simulink model "Induction_Machine_Model1"  (Simulink 7.5)
settings: Solver=ode45  StartTime=0.0  StopTime=0.2  MaxStep=0.001  RelTol=1e-3
settings Model: Creator=CN  LastModifiedBy=pradhyumna
settings DebuggingCC: StrictBusMsg=Warning

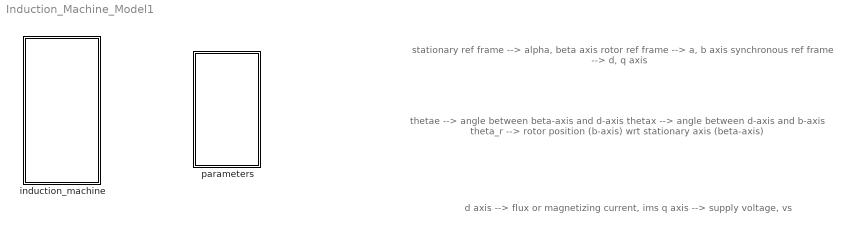
== system Induction_Machine_Model1 ==
  note: thetae --> angle between beta-axis and d-axis
      | thetax --> angle between d-axis and b-axis
      | theta_r --> rotor position (b-axis) wrt stationary axis (beta-axis)
  note: stationary ref frame --> alpha, beta axis
      | rotor ref frame --> a, b axis
      | synchronous ref frame --> d, q axis
  note: d axis --> flux or magnetizing current, ims
      | q axis --> supply voltage, vs
  induction_machine : Subsystem
  parameters : Subsystem

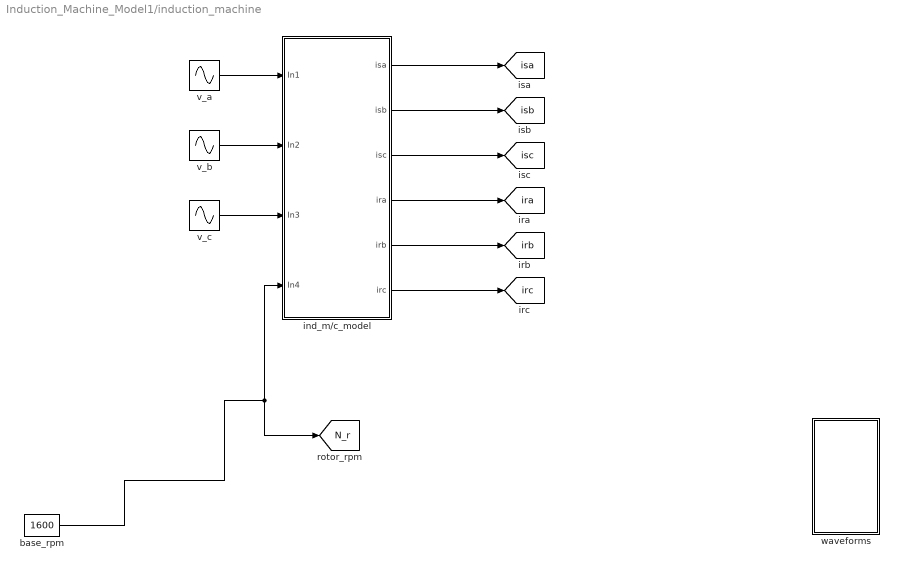
== system Induction_Machine_Model1/induction_machine ==
  base_rpm : Constant  Value=1600  OutDataType=sfix(16)  OutScaling=2^0
  ind_m/c_model : Subsystem
  v_a : Sin  Amplitude=239.6*sqrt(2)  Bias=0  Frequency=2*pi*50  Phase=0  Samples=10  SampleTime=0  Offset=0
  v_b : Sin  Amplitude=239.6*sqrt(2)  Bias=0  Frequency=2*pi*50  Phase=-2*pi/3  Samples=10  SampleTime=0  Offset=0
  v_c : Sin  Amplitude=239.6*sqrt(2)  Bias=0  Frequency=2*pi*50  Phase=-4*pi/3  Samples=10  SampleTime=0  Offset=0
  waveforms : Subsystem
  tag scope: N_r=global, ira=global, irb=global, irc=global, isa=global, isb=global, isc=global
  wires:
  ind_m/c_model/6(irc) -> [irc]
  ind_m/c_model/5(irb) -> [irb]
  ind_m/c_model/4(ira) -> [ira]
  ind_m/c_model/3(isc) -> [isc]
  ind_m/c_model/2(isb) -> [isb]
  ind_m/c_model/1(isa) -> [isa]
  v_c/1 -> ind_m/c_model/3(In3)
  v_b/1 -> ind_m/c_model/2(In2)
  v_a/1 -> ind_m/c_model/1(In1)
  base_rpm/1 -> ind_m/c_model/4(In4), [N_r]

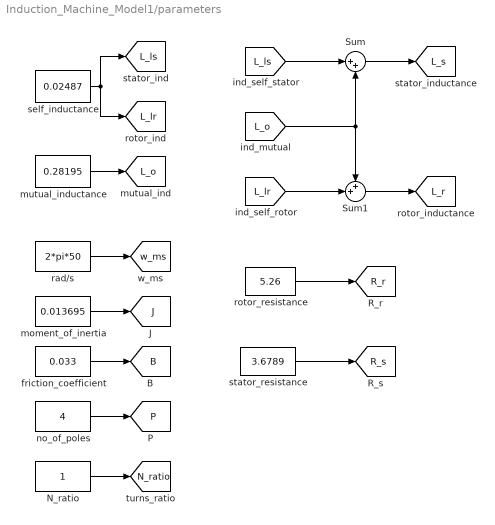
== system Induction_Machine_Model1/parameters ==
  N_ratio : Constant  OutDataType=sfix(16)  OutScaling=2^0
  Sum : Sum  Inputs=|++  OutDataType=sfix(16)  OutScaling=2^0
  Sum1 : Sum  Inputs=++|  OutDataType=sfix(16)  OutScaling=2^0
  friction_coefficient : Constant  Value=0.033  OutDataType=sfix(16)  OutScaling=2^0
  moment_of_inertia : Constant  Value=0.013695  OutDataType=sfix(16)  OutScaling=2^0
  mutual_inductance : Constant  Value=0.28195  OutDataType=sfix(16)  OutScaling=2^0
  no_of_poles : Constant  Value=4  OutDataType=sfix(16)  OutScaling=2^0
  rad/s : Constant  Value=2*pi*50  OutDataType=sfix(16)  OutScaling=2^0
  rotor_resistance : Constant  Value=5.26  OutDataType=sfix(16)  OutScaling=2^0
  self_inductance : Constant  Value=0.02487  OutDataType=sfix(16)  OutScaling=2^0
  stator_resistance : Constant  Value=3.6789  OutDataType=sfix(16)  OutScaling=2^0
  tag scope: B=global, J=global, L_lr=global, L_ls=global, L_o=global, L_r=global, L_s=global, N_ratio=global, P=global, R_r=global, R_s=global, w_ms=global
  wires:
  self_inductance/1 -> [L_ls], [L_lr]
  rad/s/1 -> [w_ms]
  moment_of_inertia/1 -> [J]
  friction_coefficient/1 -> [B]
  no_of_poles/1 -> [P]
  N_ratio/1 -> [N_ratio]
  [L_lr] -> Sum1/2
  [L_ls] -> Sum/1
  Sum/1 -> [L_s]
  Sum1/1 -> [L_r]
  rotor_resistance/1 -> [R_r]
  mutual_inductance/1 -> [L_o]
  stator_resistance/1 -> [R_s]
  [L_o] -> Sum/2, Sum1/1

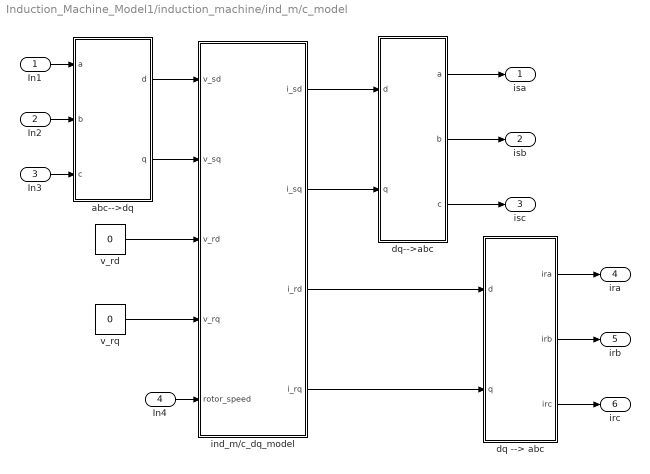
== system Induction_Machine_Model1/induction_machine/ind_m/c_model ==
  In1 : Inport  OutDataType=sfix(16)  OutScaling=2^0
  In2 : Inport  Port=2  OutDataType=sfix(16)  OutScaling=2^0
  In3 : Inport  Port=3  OutDataType=sfix(16)  OutScaling=2^0
  In4 : Inport  Port=4  OutDataType=sfix(16)  OutScaling=2^0
  abc-->dq : Subsystem
  dq --> abc : Subsystem
  dq-->abc : Subsystem
  ind_m/c_dq_model : Subsystem
  v_rd : Constant  Value=0  OutDataType=fixdt(1, 16)  OutScaling=2^0
  v_rq : Constant  Value=0  OutDataType=fixdt(1, 16)  OutScaling=2^0
  isa : Outport  OutDataType=sfix(16)  OutScaling=2^0
  isb : Outport  Port=2  OutDataType=sfix(16)  OutScaling=2^0
  isc : Outport  Port=3  OutDataType=sfix(16)  OutScaling=2^0
  ira : Outport  Port=4  OutDataType=sfix(16)  OutScaling=2^0
  irb : Outport  Port=5  OutDataType=sfix(16)  OutScaling=2^0
  irc : Outport  Port=6  OutDataType=sfix(16)  OutScaling=2^0
  wires:
  ind_m/c_dq_model/1(i_sd) -> dq-->abc/1(d)
  ind_m/c_dq_model/2(i_sq) -> dq-->abc/2(q)
  abc-->dq/2(q) -> ind_m/c_dq_model/2(v_sq)
  abc-->dq/1(d) -> ind_m/c_dq_model/1(v_sd)
  ind_m/c_dq_model/3(i_rd) -> dq --> abc/1(d)
  ind_m/c_dq_model/4(i_rq) -> dq --> abc/2(q)
  In1/1 -> abc-->dq/1(a)
  dq-->abc/1(a) -> isa/1
  In2/1 -> abc-->dq/2(b)
  dq-->abc/2(b) -> isb/1
  In3/1 -> abc-->dq/3(c)
  dq-->abc/3(c) -> isc/1
  dq --> abc/1(ira) -> ira/1
  dq --> abc/2(irb) -> irb/1
  dq --> abc/3(irc) -> irc/1
  In4/1 -> ind_m/c_dq_model/5(rotor_speed)
  v_rd/1 -> ind_m/c_dq_model/3(v_rd)
  v_rq/1 -> ind_m/c_dq_model/4(v_rq)

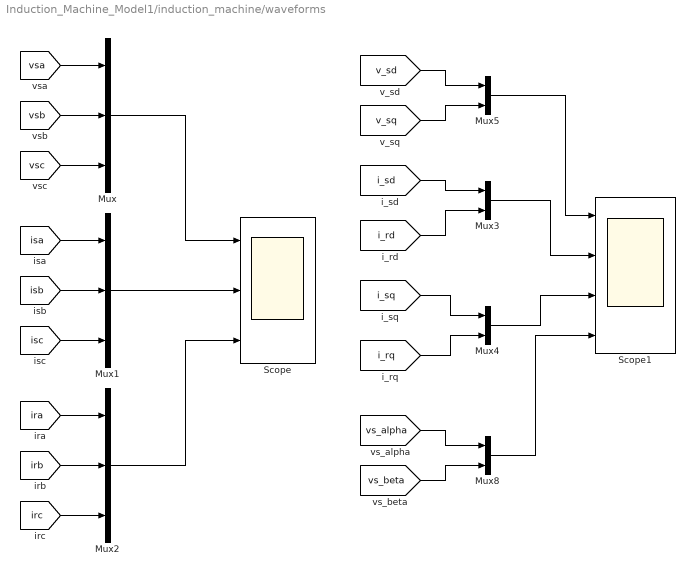
== system Induction_Machine_Model1/induction_machine/waveforms ==
  Mux : Mux  Inputs=3
  Mux1 : Mux  Inputs=3
  Mux2 : Mux  Inputs=3
  Mux{3..5,8} (4 alike) : Mux  Inputs=2
  Scope : Scope  NumInputPorts=3
      settings: TimeRange=3  YMin=-7460~-5~-5  YMax=-7390~5~5  SampleInput=on  SampleTime=0.00001
  Scope1 : Scope  NumInputPorts=4
      settings: TimeRange=3  YMin=-25~-0.5~-3~-350  YMax=350~4~3~350  SaveName=ScopeData2  SampleInput=on  SampleTime=0.00001
  wires:
  [vsa] -> Mux/1
  [vsb] -> Mux/2
  [vsc] -> Mux/3
  [isa] -> Mux1/1
  [isb] -> Mux1/2
  [isc] -> Mux1/3
  [ira] -> Mux2/1
  [irb] -> Mux2/2
  [irc] -> Mux2/3
  Mux/1 -> Scope/1
  Mux1/1 -> Scope/2
  Mux2/1 -> Scope/3
  [i_sd] -> Mux3/1
  [i_rd] -> Mux3/2
  [i_sq] -> Mux4/1
  [i_rq] -> Mux4/2
  [v_sd] -> Mux5/1
  [v_sq] -> Mux5/2
  Mux5/1 -> Scope1/1
  Mux3/1 -> Scope1/2
  Mux4/1 -> Scope1/3
  [vs_alpha] -> Mux8/1
  [vs_beta] -> Mux8/2
  Mux8/1 -> Scope1/4

== system Induction_Machine_Model1/induction_machine/ind_m/c_model/abc-->dq ==
  a : Inport  OutDataType=sfix(16)  OutScaling=2^0
  b : Inport  Port=2  OutDataType=sfix(16)  OutScaling=2^0
  c : Inport  Port=3  OutDataType=sfix(16)  OutScaling=2^0
  Subsystem : Subsystem
  d : Outport  OutDataType=sfix(16)  OutScaling=2^0
  q : Outport  Port=2  OutDataType=sfix(16)  OutScaling=2^0
  tag scope: v_sd=global, v_sq=global, vsa=global, vsb=global, vsc=global
  wires:
  a/1 -> [vsa], Subsystem/1(a)
  Subsystem/1(d) -> d/1, [v_sd]
  b/1 -> [vsb], Subsystem/2(b)
  Subsystem/2(q) -> q/1, [v_sq]
  c/1 -> [vsc], Subsystem/3(c)

== system Induction_Machine_Model1/induction_machine/ind_m/c_model/dq --> abc ==
  d : Inport  OutDataType=sfix(16)  OutScaling=2^0
  q : Inport  Port=2  OutDataType=sfix(16)  OutScaling=2^0
  ab-->abc : Subsystem
  dq-->ab : Subsystem
  ira : Outport  OutDataType=sfix(16)  OutScaling=2^0
  irb : Outport  Port=2  OutDataType=sfix(16)  OutScaling=2^0
  irc : Outport  Port=3  OutDataType=sfix(16)  OutScaling=2^0
  wires:
  dq-->ab/1(ir_a) -> ab-->abc/1(ir_a)
  dq-->ab/2(ir_b) -> ab-->abc/2(ir_b)
  ab-->abc/1(a) -> ira/1
  d/1 -> dq-->ab/1(ird)
  ab-->abc/2(b) -> irb/1
  q/1 -> dq-->ab/2(irq)
  ab-->abc/3(c) -> irc/1

== system Induction_Machine_Model1/induction_machine/ind_m/c_model/dq-->abc ==
  d : Inport  OutDataType=sfix(16)  OutScaling=2^0
  q : Inport  Port=2  OutDataType=sfix(16)  OutScaling=2^0
  alpha-->abc : Subsystem
  dq-->alpha : Subsystem
  a : Outport  OutDataType=sfix(16)  OutScaling=2^0
  b : Outport  Port=2  OutDataType=sfix(16)  OutScaling=2^0
  c : Outport  Port=3  OutDataType=sfix(16)  OutScaling=2^0
  wires:
  dq-->alpha/1(alpha) -> alpha-->abc/1(alpha)
  dq-->alpha/2(beta) -> alpha-->abc/2(beta)
  alpha-->abc/1(a) -> a/1
  d/1 -> dq-->alpha/1(d)
  alpha-->abc/2(b) -> b/1
  q/1 -> dq-->alpha/2(q)
  alpha-->abc/3(c) -> c/1

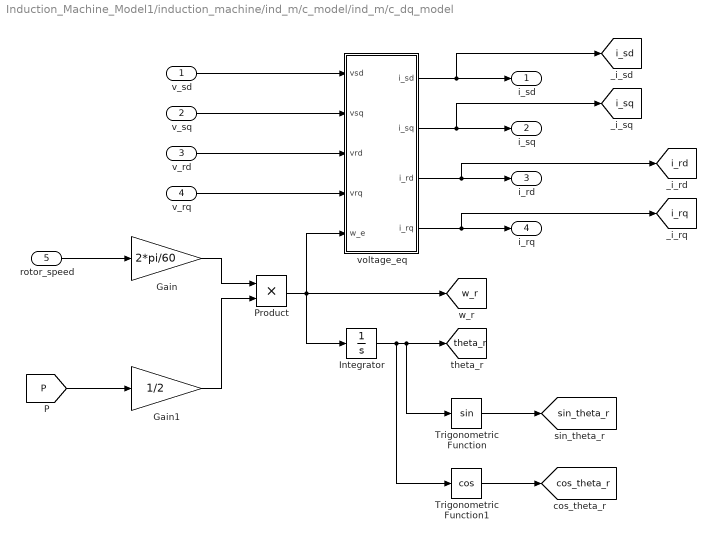
== system Induction_Machine_Model1/induction_machine/ind_m/c_model/ind_m/c_dq_model ==
  v_sd : Inport  OutDataType=sfix(16)  OutScaling=2^0
  v_sq : Inport  Port=2  OutDataType=sfix(16)  OutScaling=2^0
  v_rd : Inport  Port=3  OutDataType=sfix(16)  OutScaling=2^0
  v_rq : Inport  Port=4  OutDataType=sfix(16)  OutScaling=2^0
  rotor_speed : Inport  Port=5  OutDataType=sfix(16)  OutScaling=2^0
  Gain : Gain  Gain=2*pi/60  ParameterDataType=sfix(16)  ParameterScaling=2^0  OutDataType=sfix(16)  OutScaling=2^0
  Gain1 : Gain  Gain=1/2  ParameterDataType=sfix(16)  ParameterScaling=2^0  OutDataType=sfix(16)  OutScaling=2^0
  Integrator : Integrator
  Product : Product  OutDataType=sfix(16)  OutScaling=2^0  RndMeth=Zero
  Trigonometric Function : Trigonometry
  Trigonometric Function1 : Trigonometry  Operator=cos
  voltage_eq : Subsystem
  i_sd : Outport  OutDataType=sfix(16)  OutScaling=2^0
  i_sq : Outport  Port=2  OutDataType=sfix(16)  OutScaling=2^0
  i_rd : Outport  Port=3  OutDataType=sfix(16)  OutScaling=2^0
  i_rq : Outport  Port=4  OutDataType=sfix(16)  OutScaling=2^0
  tag scope: cos_theta_r=global, i_rd=global, i_rq=global, i_sd=global, i_sq=global, sin_theta_r=global, theta_r=global, w_r=global
  wires:
  v_sd/1 -> voltage_eq/1(vsd)
  v_sq/1 -> voltage_eq/2(vsq)
  v_rd/1 -> voltage_eq/3(vrd)
  v_rq/1 -> voltage_eq/4(vrq)
  voltage_eq/1(i_sd) -> i_sd/1, [i_sd]
  voltage_eq/2(i_sq) -> i_sq/1, [i_sq]
  voltage_eq/3(i_rd) -> i_rd/1, [i_rd]
  voltage_eq/4(i_rq) -> i_rq/1, [i_rq]
  rotor_speed/1 -> Gain/1
  Gain/1 -> Product/1
  [P] -> Gain1/1
  Gain1/1 -> Product/2
  Product/1 -> Integrator/1, voltage_eq/5(w_e), [w_r]
  Integrator/1 -> [theta_r], Trigonometric Function/1, Trigonometric Function1/1
  Trigonometric Function/1 -> [sin_theta_r]
  Trigonometric Function1/1 -> [cos_theta_r]

== system Induction_Machine_Model1/induction_machine/ind_m/c_model/abc-->dq/Subsystem ==
  a : Inport
  b : Inport  Port=2
  c : Inport  Port=3
  Mux : Mux  Inputs=2
  abc-->alpha : Subsystem
  alpha-->dq : Subsystem
  cos_cal : Fcn  Expr=u(1)/sqrt(u(1)^2+u(2)^2)
  sin_cal : Fcn  Expr=-u(2)/sqrt(u(1)^2+u(2)^2)
  d : Outport
  q : Outport  Port=2
  tag scope: cos_thetae=global, sin_thetae=global
  wires:
  abc-->alpha/2(beta) -> alpha-->dq/2(beta), Mux/2
  abc-->alpha/1(alpha) -> alpha-->dq/1(alpha), Mux/1
  Mux/1 -> sin_cal/1, cos_cal/1
  sin_cal/1 -> [sin_thetae]
  cos_cal/1 -> [cos_thetae]
  a/1 -> abc-->alpha/1(a)
  b/1 -> abc-->alpha/2(b)
  c/1 -> abc-->alpha/3(c)
  alpha-->dq/1(d) -> d/1
  alpha-->dq/2(q) -> q/1

== system Induction_Machine_Model1/induction_machine/ind_m/c_model/dq --> abc/ab-->abc ==
  ir_a : Inport  OutDataType=sfix(16)  OutScaling=2^0
  ir_b : Inport  Port=2  OutDataType=sfix(16)  OutScaling=2^0
  Fcn : Fcn  Expr=u(1)
  Fcn1 : Fcn  Expr=-u(1)/2-u(2)*sqrt(3)/2
  Fcn2 : Fcn  Expr=-u(1)/2+u(2)*sqrt(3)/2
  Mux : Mux  Inputs=2
  a : Outport  OutDataType=sfix(16)  OutScaling=2^0
  b : Outport  Port=2  OutDataType=sfix(16)  OutScaling=2^0
  c : Outport  Port=3  OutDataType=sfix(16)  OutScaling=2^0
  wires:
  Mux/1 -> Fcn/1, Fcn1/1, Fcn2/1
  Fcn/1 -> a/1
  Fcn1/1 -> b/1
  Fcn2/1 -> c/1
  ir_a/1 -> Mux/1
  ir_b/1 -> Mux/2

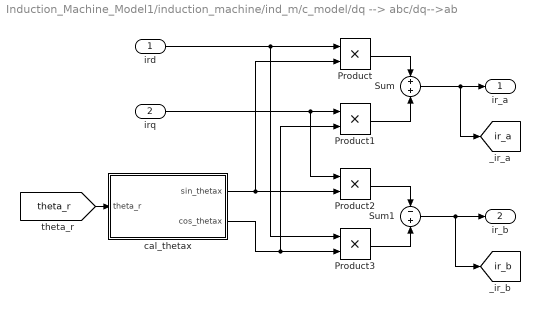
== system Induction_Machine_Model1/induction_machine/ind_m/c_model/dq --> abc/dq-->ab ==
  ird : Inport  OutDataType=sfix(16)  OutScaling=2^0
  irq : Inport  Port=2  OutDataType=sfix(16)  OutScaling=2^0
  Product{,1..3} (4 alike) : Product  OutDataType=sfix(16)  OutScaling=2^0  RndMeth=Zero
  Sum : Sum  OutDataType=sfix(16)  OutScaling=2^0
  Sum1 : Sum  Inputs=-+  OutDataType=sfix(16)  OutScaling=2^0
  cal_thetax : Subsystem
  ir_a : Outport  OutDataType=sfix(16)  OutScaling=2^0
  ir_b : Outport  Port=2  OutDataType=sfix(16)  OutScaling=2^0
  tag scope: ir_a=global, ir_b=global
  wires:
  [theta_r] -> cal_thetax/1(theta_r)
  ird/1 -> Product3/1, Product/1
  cal_thetax/1(sin_thetax) -> Product/2, Product2/2
  irq/1 -> Product2/1, Product1/1
  cal_thetax/2(cos_thetax) -> Product1/2, Product3/2
  Product/1 -> Sum/1
  Product1/1 -> Sum/2
  Product2/1 -> Sum1/1
  Product3/1 -> Sum1/2
  Sum/1 -> ir_a/1, [ir_a]
  Sum1/1 -> ir_b/1, [ir_b]

== system Induction_Machine_Model1/induction_machine/ind_m/c_model/dq-->abc/alpha-->abc ==
  alpha : Inport  OutDataType=sfix(16)  OutScaling=2^0
  beta : Inport  Port=2  OutDataType=sfix(16)  OutScaling=2^0
  Fcn : Fcn  Expr=u(1)
  Fcn1 : Fcn  Expr=-u(1)/2-u(2)*sqrt(3)/2
  Fcn2 : Fcn  Expr=-u(1)/2+u(2)*sqrt(3)/2
  Mux : Mux  Inputs=2
  a : Outport  OutDataType=sfix(16)  OutScaling=2^0
  b : Outport  Port=2  OutDataType=sfix(16)  OutScaling=2^0
  c : Outport  Port=3  OutDataType=sfix(16)  OutScaling=2^0
  wires:
  Mux/1 -> Fcn/1, Fcn1/1, Fcn2/1
  Fcn/1 -> a/1
  Fcn1/1 -> b/1
  Fcn2/1 -> c/1
  alpha/1 -> Mux/1
  beta/1 -> Mux/2

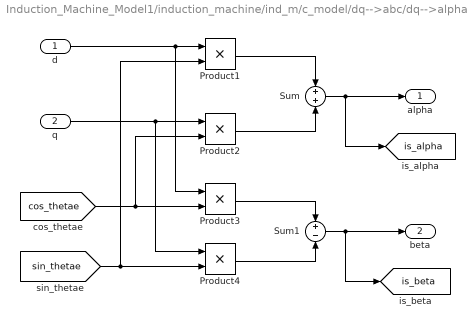
== system Induction_Machine_Model1/induction_machine/ind_m/c_model/dq-->abc/dq-->alpha ==
  d : Inport  OutDataType=sfix(16)  OutScaling=2^0
  q : Inport  Port=2  OutDataType=sfix(16)  OutScaling=2^0
  Product{1..4} (4 alike) : Product  OutDataType=sfix(16)  OutScaling=2^0  RndMeth=Zero
  Sum : Sum  OutDataType=sfix(16)  OutScaling=2^0
  Sum1 : Sum  Inputs=+-  OutDataType=sfix(16)  OutScaling=2^0
  alpha : Outport  OutDataType=sfix(16)  OutScaling=2^0
  beta : Outport  Port=2  OutDataType=sfix(16)  OutScaling=2^0
  tag scope: is_alpha=global, is_beta=global
  wires:
  d/1 -> Product1/1, Product3/1
  q/1 -> Product2/1, Product4/1
  [cos_thetae] -> Product3/2, Product2/2
  [sin_thetae] -> Product4/2, Product1/2
  Product1/1 -> Sum/1
  Product2/1 -> Sum/2
  Product3/1 -> Sum1/1
  Product4/1 -> Sum1/2
  Sum/1 -> alpha/1, [is_alpha]
  Sum1/1 -> beta/1, [is_beta]

== system Induction_Machine_Model1/induction_machine/ind_m/c_model/ind_m/c_dq_model/voltage_eq ==
  vsd : Inport  OutDataType=sfix(16)  OutScaling=2^0
  vsq : Inport  Port=2  OutDataType=sfix(16)  OutScaling=2^0
  vrd : Inport  Port=3  OutDataType=sfix(16)  OutScaling=2^0
  vrq : Inport  Port=4  OutDataType=sfix(16)  OutScaling=2^0
  w_e : Inport  Port=5  OutDataType=sfix(16)  OutScaling=2^0
  rotor_d_eq : Subsystem
  rotor_q_eq : Subsystem
  stator_d_eq : Subsystem
  stator_q_eq : Subsystem
  i_sd : Outport  OutDataType=sfix(16)  OutScaling=2^0
  i_sq : Outport  Port=2  OutDataType=sfix(16)  OutScaling=2^0
  i_rd : Outport  Port=3  OutDataType=sfix(16)  OutScaling=2^0
  i_rq : Outport  Port=4  OutDataType=sfix(16)  OutScaling=2^0
  wires:
  stator_d_eq/1(i_sd) -> rotor_q_eq/2(isd), rotor_d_eq/2(isd), stator_q_eq/2(isd), stator_d_eq/2(isd), i_sd/1
  stator_q_eq/1(i_sq) -> stator_d_eq/3(isq), rotor_q_eq/3(isq), rotor_d_eq/3(isq), stator_q_eq/3(isq), i_sq/1
  rotor_d_eq/1(i_rd) -> stator_d_eq/4("ird\""), stator_q_eq/4("ird\""), rotor_q_eq/4("ird\""), rotor_d_eq/4("ird\""), i_rd/1
  rotor_q_eq/1(i_rq) -> stator_d_eq/5("irq\""), stator_q_eq/5("irq\""), rotor_d_eq/5("irq\""), rotor_q_eq/5("irq\""), i_rq/1
  w_e/1 -> rotor_q_eq/6(w_e), rotor_d_eq/6(w_e)
  vsd/1 -> stator_d_eq/1(v_sd)
  vsq/1 -> stator_q_eq/1(v_sq)
  vrd/1 -> rotor_d_eq/1(v_rd)
  vrq/1 -> rotor_q_eq/1(v_rq)

== system Induction_Machine_Model1/induction_machine/ind_m/c_model/abc-->dq/Subsystem/abc-->alpha ==
  a : Inport  OutDataType=sfix(16)  OutScaling=2^0
  b : Inport  Port=2  OutDataType=sfix(16)  OutScaling=2^0
  c : Inport  Port=3  OutDataType=sfix(16)  OutScaling=2^0
  Mux : Mux  Inputs=3
  alpha_cal : Fcn  Expr=2/3*(u(1)+u(2)*cos(-2*pi/3)+u(3)*cos(-4*pi/3))
  beta_cal : Fcn  Expr=2/3*(u(2)*sin(-2*pi/3)+u(3)*sin(-4*pi/3))
  alpha : Outport  OutDataType=sfix(16)  OutScaling=2^0
  beta : Outport  Port=2  OutDataType=sfix(16)  OutScaling=2^0
  tag scope: vs_alpha=global, vs_beta=global
  wires:
  Mux/1 -> alpha_cal/1, beta_cal/1
  a/1 -> Mux/1
  alpha_cal/1 -> alpha/1, [vs_alpha]
  b/1 -> Mux/2
  beta_cal/1 -> beta/1, [vs_beta]
  c/1 -> Mux/3

== system Induction_Machine_Model1/induction_machine/ind_m/c_model/abc-->dq/Subsystem/alpha-->dq ==
  alpha : Inport  OutDataType=sfix(16)  OutScaling=2^0
  beta : Inport  Port=2  OutDataType=sfix(16)  OutScaling=2^0
  Product{1..4} (4 alike) : Product  OutDataType=sfix(16)  OutScaling=2^0  RndMeth=Zero
  Sum : Sum  OutDataType=sfix(16)  OutScaling=2^0
  Sum1 : Sum  Inputs=+-  OutDataType=sfix(16)  OutScaling=2^0
  d : Outport  OutDataType=sfix(16)  OutScaling=2^0
  q : Outport  Port=2  OutDataType=sfix(16)  OutScaling=2^0
  wires:
  alpha/1 -> Product3/1, Product1/1
  beta/1 -> Product4/1, Product2/1
  [cos_thetae] -> Product3/2, Product2/2
  [sin_thetae] -> Product4/2, Product1/2
  Product1/1 -> Sum/1
  Product2/1 -> Sum/2
  Product3/1 -> Sum1/1
  Product4/1 -> Sum1/2
  Sum/1 -> d/1
  Sum1/1 -> q/1

== system Induction_Machine_Model1/induction_machine/ind_m/c_model/dq --> abc/dq-->ab/cal_thetax ==
  theta_r : Inport  OutDataType=sfix(16)  OutScaling=2^0
  Product{,1..3} (4 alike) : Product  OutDataType=sfix(16)  OutScaling=2^0  RndMeth=Zero
  Sum : Sum  Inputs=+-  OutDataType=sfix(16)  OutScaling=2^0
  Sum1 : Sum  OutDataType=sfix(16)  OutScaling=2^0
  cos_thetar : Trigonometry  Operator=cos
  sin_thetar : Trigonometry
  sin_thetax : Outport  OutDataType=sfix(16)  OutScaling=2^0
  cos_thetax : Outport  Port=2  OutDataType=sfix(16)  OutScaling=2^0
  wires:
  theta_r/1 -> cos_thetar/1, sin_thetar/1
  [sin_thetae] -> Product/1, Product2/1
  cos_thetar/1 -> Product/2, Product3/2
  [cos_thetae] -> Product1/1, Product3/1
  sin_thetar/1 -> Product1/2, Product2/2
  Product/1 -> Sum/1
  Product1/1 -> Sum/2
  Product2/1 -> Sum1/1
  Product3/1 -> Sum1/2
  Sum/1 -> sin_thetax/1
  Sum1/1 -> cos_thetax/1

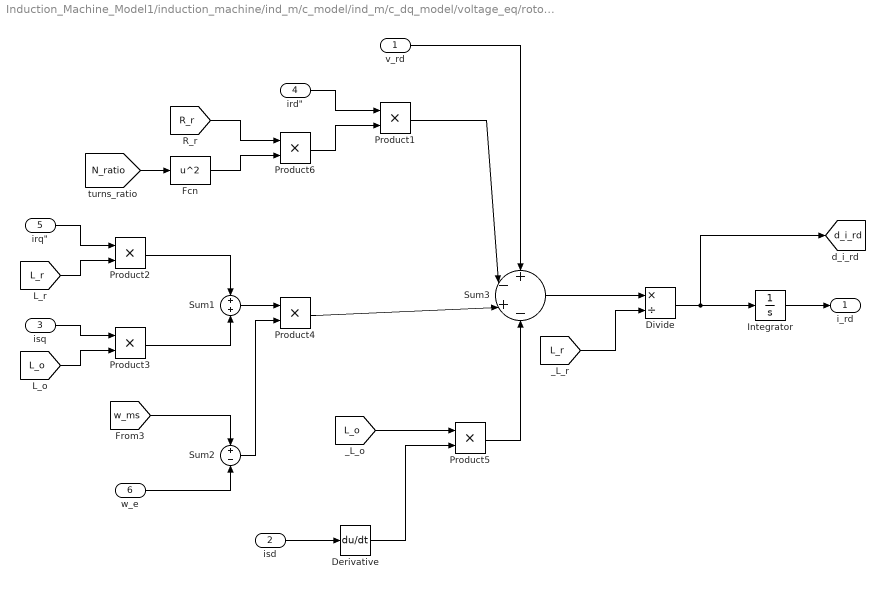
== system Induction_Machine_Model1/induction_machine/ind_m/c_model/ind_m/c_dq_model/voltage_eq/rotor_d_eq ==
  v_rd : Inport  OutDataType=sfix(16)  OutScaling=2^0
  isd : Inport  Port=2  OutDataType=sfix(16)  OutScaling=2^0
  isq : Inport  Port=3  OutDataType=sfix(16)  OutScaling=2^0
  "ird\"" : Inport  Port=4  OutDataType=sfix(16)  OutScaling=2^0
  "irq\"" : Inport  Port=5  OutDataType=sfix(16)  OutScaling=2^0
  w_e : Inport  Port=6  OutDataType=sfix(16)  OutScaling=2^0
  Derivative : Derivative
  Divide : Product  Inputs=*/  OutDataType=sfix(16)  OutScaling=2^-10
  Fcn : Fcn  Expr=u^2
  Integrator : Integrator
  Product{1..6} (6 alike) : Product  OutDataType=sfix(16)  OutScaling=2^0  RndMeth=Zero
  Sum1 : Sum  OutDataType=sfix(16)  OutScaling=2^0
  Sum2 : Sum  Inputs=+-  OutDataType=sfix(16)  OutScaling=2^0
  Sum3 : Sum  Inputs=+-+-  OutDataType=sfix(16)  OutScaling=2^0
  i_rd : Outport  OutDataType=sfix(16)  OutScaling=2^0
  tag scope: d_i_rd=global
  wires:
  "ird\""/1 -> Product1/1
  "irq\""/1 -> Product2/1
  [L_r] -> Product2/2
  isq/1 -> Product3/1
  [L_o] -> Product3/2
  Product2/1 -> Sum1/1
  Product3/1 -> Sum1/2
  [w_ms] -> Sum2/1
  w_e/1 -> Sum2/2
  Sum1/1 -> Product4/1
  Sum2/1 -> Product4/2
  isd/1 -> Derivative/1
  v_rd/1 -> Sum3/1
  Product1/1 -> Sum3/2
  Product4/1 -> Sum3/3
  Product5/1 -> Sum3/4
  Sum3/1 -> Divide/1
  [L_r] -> Divide/2
  Divide/1 -> [d_i_rd], Integrator/1
  [N_ratio] -> Fcn/1
  [R_r] -> Product6/1
  Fcn/1 -> Product6/2
  Product6/1 -> Product1/2
  Integrator/1 -> i_rd/1
  [L_o] -> Product5/1
  Derivative/1 -> Product5/2

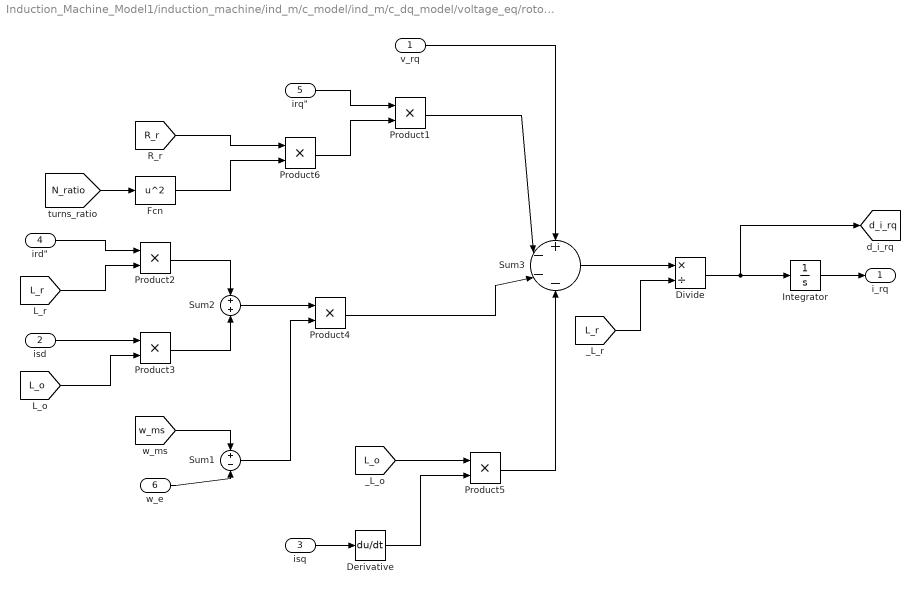
== system Induction_Machine_Model1/induction_machine/ind_m/c_model/ind_m/c_dq_model/voltage_eq/rotor_q_eq ==
  v_rq : Inport  OutDataType=sfix(16)  OutScaling=2^0
  isd : Inport  Port=2  OutDataType=sfix(16)  OutScaling=2^0
  isq : Inport  Port=3  OutDataType=sfix(16)  OutScaling=2^0
  "ird\"" : Inport  Port=4  OutDataType=sfix(16)  OutScaling=2^0
  "irq\"" : Inport  Port=5  OutDataType=sfix(16)  OutScaling=2^0
  w_e : Inport  Port=6  OutDataType=sfix(16)  OutScaling=2^0
  Derivative : Derivative
  Divide : Product  Inputs=*/  OutDataType=sfix(16)  OutScaling=2^-10
  Fcn : Fcn  Expr=u^2
  Integrator : Integrator
  Product{1..6} (6 alike) : Product  OutDataType=sfix(16)  OutScaling=2^0  RndMeth=Zero
  Sum1 : Sum  Inputs=+-  OutDataType=sfix(16)  OutScaling=2^0
  Sum2 : Sum  OutDataType=sfix(16)  OutScaling=2^0
  Sum3 : Sum  Inputs=+---  OutDataType=sfix(16)  OutScaling=2^0
  i_rq : Outport  OutDataType=sfix(16)  OutScaling=2^0
  tag scope: d_i_rq=global
  wires:
  "irq\""/1 -> Product1/1
  Product6/1 -> Product1/2
  "ird\""/1 -> Product2/1
  [L_r] -> Product2/2
  isd/1 -> Product3/1
  [L_o] -> Product3/2
  [w_ms] -> Sum1/1
  w_e/1 -> Sum1/2
  Product2/1 -> Sum2/1
  Product3/1 -> Sum2/2
  Sum2/1 -> Product4/1
  Sum1/1 -> Product4/2
  isq/1 -> Derivative/1
  v_rq/1 -> Sum3/1
  Product1/1 -> Sum3/2
  Product4/1 -> Sum3/3
  Product5/1 -> Sum3/4
  Sum3/1 -> Divide/1
  [L_r] -> Divide/2
  Divide/1 -> [d_i_rq], Integrator/1
  [N_ratio] -> Fcn/1
  [R_r] -> Product6/1
  Fcn/1 -> Product6/2
  Integrator/1 -> i_rq/1
  [L_o] -> Product5/1
  Derivative/1 -> Product5/2

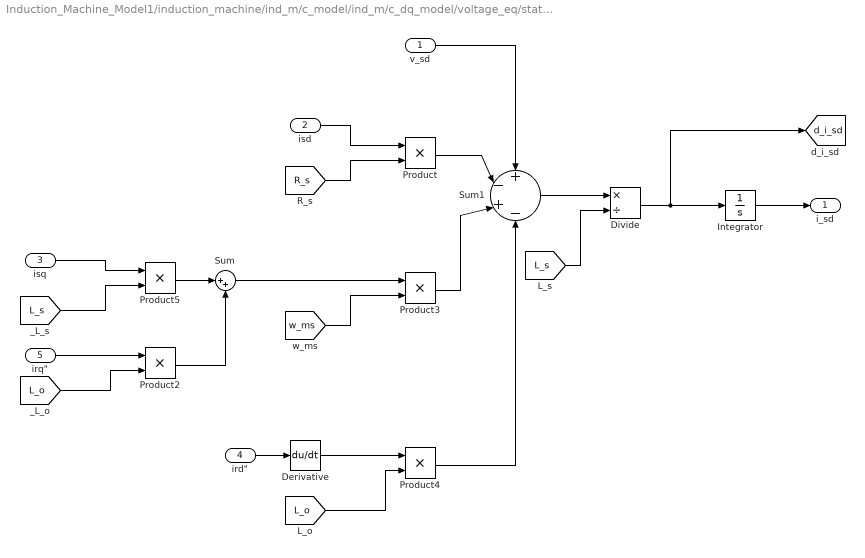
== system Induction_Machine_Model1/induction_machine/ind_m/c_model/ind_m/c_dq_model/voltage_eq/stator_d_eq ==
  v_sd : Inport  OutDataType=sfix(16)  OutScaling=2^0
  isd : Inport  Port=2  OutDataType=sfix(16)  OutScaling=2^0
  isq : Inport  Port=3  OutDataType=sfix(16)  OutScaling=2^0
  "ird\"" : Inport  Port=4  OutDataType=sfix(16)  OutScaling=2^0
  "irq\"" : Inport  Port=5  OutDataType=sfix(16)  OutScaling=2^0
  Derivative : Derivative
  Divide : Product  Inputs=*/  OutDataType=sfix(16)  OutScaling=2^-10
  Integrator : Integrator
  Product{,2..5} (5 alike) : Product  OutDataType=sfix(16)  OutScaling=2^0  RndMeth=Zero
  Sum : Sum  Inputs=|++  OutDataType=sfix(16)  OutScaling=2^0
  Sum1 : Sum  Inputs=+-+-  OutDataType=sfix(16)  OutScaling=2^0
  i_sd : Outport  OutDataType=sfix(16)  OutScaling=2^0
  tag scope: d_i_sd=global
  wires:
  isd/1 -> Product/1
  [R_s] -> Product/2
  isq/1 -> Product5/1
  [L_s] -> Product5/2
  "irq\""/1 -> Product2/1
  [L_o] -> Product2/2
  Product5/1 -> Sum/1
  Product2/1 -> Sum/2
  [w_ms] -> Product3/2
  Sum/1 -> Product3/1
  "ird\""/1 -> Derivative/1
  Derivative/1 -> Product4/1
  [L_o] -> Product4/2
  v_sd/1 -> Sum1/1
  Product/1 -> Sum1/2
  Product3/1 -> Sum1/3
  Product4/1 -> Sum1/4
  Sum1/1 -> Divide/1
  [L_s] -> Divide/2
  Divide/1 -> Integrator/1, [d_i_sd]
  Integrator/1 -> i_sd/1

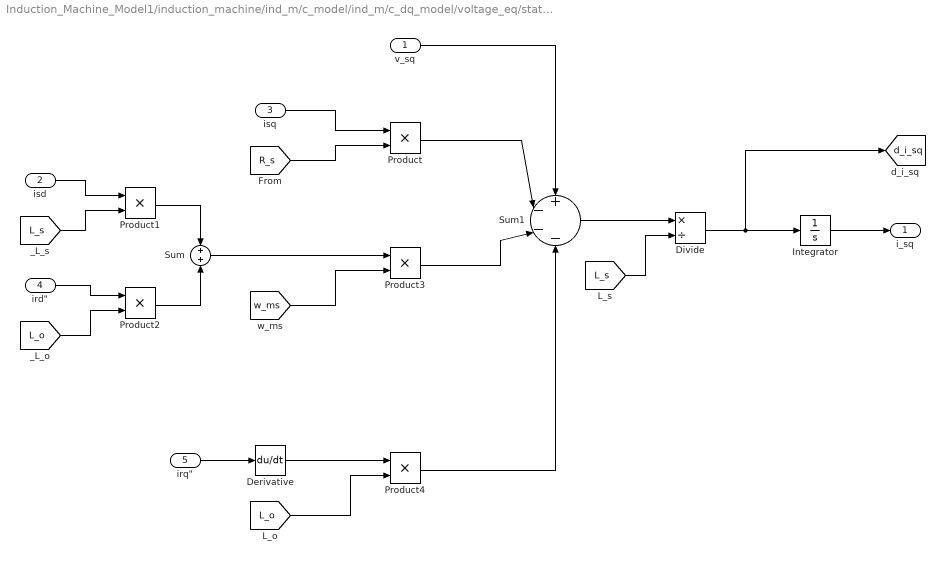
== system Induction_Machine_Model1/induction_machine/ind_m/c_model/ind_m/c_dq_model/voltage_eq/stator_q_eq ==
  v_sq : Inport  OutDataType=sfix(16)  OutScaling=2^0
  isd : Inport  Port=2  OutDataType=sfix(16)  OutScaling=2^0
  isq : Inport  Port=3  OutDataType=sfix(16)  OutScaling=2^0
  "ird\"" : Inport  Port=4  OutDataType=sfix(16)  OutScaling=2^0
  "irq\"" : Inport  Port=5  OutDataType=sfix(16)  OutScaling=2^0
  Derivative : Derivative
  Divide : Product  Inputs=*/  OutDataType=sfix(16)  OutScaling=2^-10
  Integrator : Integrator
  Product{,1..4} (5 alike) : Product  OutDataType=sfix(16)  OutScaling=2^0  RndMeth=Zero
  Sum : Sum  OutDataType=sfix(16)  OutScaling=2^0
  Sum1 : Sum  Inputs=+---  OutDataType=sfix(16)  OutScaling=2^0
  i_sq : Outport  OutDataType=sfix(16)  OutScaling=2^0
  tag scope: d_i_sq=global
  wires:
  isq/1 -> Product/1
  [R_s] -> Product/2
  isd/1 -> Product1/1
  [L_s] -> Product1/2
  "ird\""/1 -> Product2/1
  [L_o] -> Product2/2
  Product1/1 -> Sum/1
  Product2/1 -> Sum/2
  Sum/1 -> Product3/1
  "irq\""/1 -> Derivative/1
  Derivative/1 -> Product4/1
  [L_o] -> Product4/2
  v_sq/1 -> Sum1/1
  Product/1 -> Sum1/2
  Product3/1 -> Sum1/3
  Product4/1 -> Sum1/4
  Sum1/1 -> Divide/1
  [L_s] -> Divide/2
  Divide/1 -> [d_i_sq], Integrator/1
  Integrator/1 -> i_sq/1
  [w_ms] -> Product3/2
